simulink model "hex_simplify_control"  (R2017a)
settings: Solver=VariableStepAuto  StartTime=0.0  StopTime=2  RelTol=1e-3
model workspace: external: MATLAB File C:\Users\laure\Documents\Gonzalo\Robotica-II\hexapod-robot\simscape\simplify_model\hex_DataFile1.m (data not in the file)
undefined symbols (not defined in the file): qdd_1, qdd_2, qdd_3, sample_frequency, smiData, X, Y, Z
libraries: sm_lib x20, nesl_utility x19
settings Model: Creator=laure  LastModifiedBy=laure

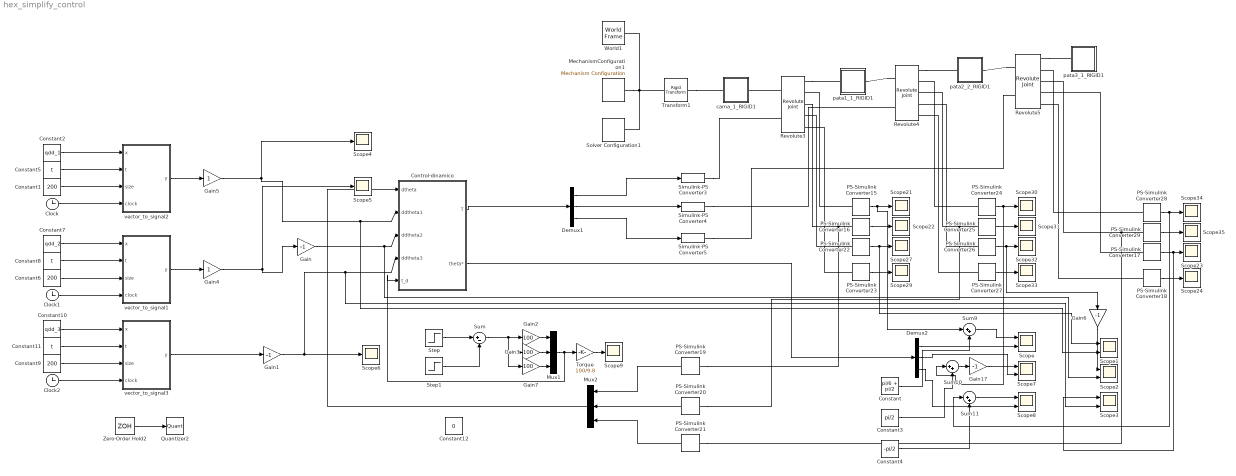
== system hex_simplify_control ==
  Clock : Clock
  Clock1 : Clock
  Clock2 : Clock
  Constant : Constant  Value=pi/6 + pi/2
  Constant1 : Constant  Value=200
  Constant10 : Constant  Value=qdd_3
  Constant11 : Constant  Value=t
  Constant12 : Constant  Value=0
  Constant2 : Constant  Value=qdd_1
  Constant3 : Constant  Value=pi/2
  Constant4 : Constant  Value=-pi/2
  Constant5 : Constant  Value=t
  Constant6 : Constant  Value=200
  Constant7 : Constant  Value=qdd_2
  Constant8 : Constant  Value=t
  Constant9 : Constant  Value=200
  Control-dinamico : Subsystem
  Demux1 : Demux  Outputs=3
  Demux2 : Demux  Outputs=3
  Gain{,1,6,17} (4 alike) : Gain  Gain=-1
  Gain2 : Gain  Gain=100
  Gain3 : Gain  Gain=100
  Gain4 : Gain
  Gain5 : Gain
  Gain7 : Gain  Gain=100
  MechanismConfiguration1 : sm_lib/Utilities/Mechanism Configuration  UniformGravity=Constant  GravityVector=[0 0 -9.81]  GravityUnits=m/s^2  LinearizationDelta=0.001
  Mux1 : Mux  Inputs=3
  Mux2 : Mux  Inputs=3
  PS-Simulink Converter{15..29} (15 alike) : nesl_utility/PS-Simulink Converter  PhysicalDomain=network_engine_domain  SubClassName=ps_output  LeftPortType=input  RightPortType=output  PseudoPeriodic=off  Frequencies=[]  Unit=1  AffineConversion=off
  Quantizer2 : Quantizer  QuantizationInterval=1/sample_frequency
  Revolute3 : sm_lib/Joints/Revolute Joint  SenseConstraintForce=off  SenseConstraintForceX=off  SenseConstraintForceY=off  SenseConstraintForceZ=off  SenseConstraintTorque=off  SenseConstraintTorqueX=off  SenseConstraintTorqueY=off  SenseConstraintTorqueZ=off  SenseTotalForce=off  SenseTotalForceX=off  SenseTotalForceY=off  SenseTotalForceZ=off  SenseTotalTorque=off  SenseTotalTorqueX=off  SenseTotalTorqueY=off  SenseTotalTorqueZ=off  CompositeWrenchDir=FollowerOnBase  CompositeWrenchFrame=BaseFrame  EquilibriumPosition=0  EquilibriumPositionUnits=rad  SpringStiffness=0  SpringStiffnessUnits=N*m/rad  DampingCoefficient=0.1  DampingCoefficientUnits=N*m/(rad/s)  TorqueActuationMode=InputTorque  MotionActuationMode=ComputedMotion  SensePosition=on  SenseVelocity=on  SenseAcceleration=on  SenseTorqueForce=on  PositionTargetSpecify=on  PositionTargetPriority=Low  PositionTargetValue=-pi/2 - pi/6  PositionTargetValueUnits=rad  VelocityTargetSpecify=off  VelocityTargetPriority=High  VelocityTargetValue=0  VelocityTargetValueUnits=deg/s
  Revolute4 : sm_lib/Joints/Revolute Joint  SenseConstraintForce=off  SenseConstraintForceX=off  SenseConstraintForceY=off  SenseConstraintForceZ=off  SenseConstraintTorque=off  SenseConstraintTorqueX=off  SenseConstraintTorqueY=off  SenseConstraintTorqueZ=off  SenseTotalForce=off  SenseTotalForceX=off  SenseTotalForceY=off  SenseTotalForceZ=off  SenseTotalTorque=off  SenseTotalTorqueX=off  SenseTotalTorqueY=off  SenseTotalTorqueZ=off  CompositeWrenchDir=FollowerOnBase  CompositeWrenchFrame=BaseFrame  EquilibriumPosition=0  EquilibriumPositionUnits=rad  SpringStiffness=0  SpringStiffnessUnits=N*m/rad  DampingCoefficient=0.1  DampingCoefficientUnits=N*m/(rad/s)  TorqueActuationMode=InputTorque  MotionActuationMode=ComputedMotion  SensePosition=on  SenseVelocity=on  SenseAcceleration=on  SenseTorqueForce=on  PositionTargetSpecify=on  PositionTargetPriority=Low  PositionTargetValue=-pi/2  PositionTargetValueUnits=rad  VelocityTargetSpecify=on  VelocityTargetPriority=High  VelocityTargetValue=0  VelocityTargetValueUnits=deg/s
  Revolute5 : sm_lib/Joints/Revolute Joint  SenseConstraintForce=off  SenseConstraintForceX=off  SenseConstraintForceY=off  SenseConstraintForceZ=off  SenseConstraintTorque=off  SenseConstraintTorqueX=off  SenseConstraintTorqueY=off  SenseConstraintTorqueZ=off  SenseTotalForce=off  SenseTotalForceX=off  SenseTotalForceY=off  SenseTotalForceZ=off  SenseTotalTorque=off  SenseTotalTorqueX=off  SenseTotalTorqueY=off  SenseTotalTorqueZ=off  CompositeWrenchDir=FollowerOnBase  CompositeWrenchFrame=BaseFrame  EquilibriumPosition=0  EquilibriumPositionUnits=rad  SpringStiffness=0  SpringStiffnessUnits=N*m/rad  DampingCoefficient=0.1  DampingCoefficientUnits=N*m/(rad/s)  TorqueActuationMode=InputTorque  MotionActuationMode=ComputedMotion  SensePosition=on  SenseVelocity=on  SenseAcceleration=on  SenseTorqueForce=on  PositionTargetSpecify=on  PositionTargetPriority=Low  PositionTargetValue=0  PositionTargetValueUnits=rad  VelocityTargetSpecify=off  VelocityTargetPriority=High  VelocityTargetValue=0  VelocityTargetValueUnits=deg/s
  Scope{,1..3,7..8} (6 alike) : Scope  NumInputPorts=2
  Scope{4..6,9,21..24,27,29..35} (16 alike) : Scope
  Simulink-PS Converter3 : nesl_utility/Simulink-PS Converter  PhysicalDomain=network_engine_domain  SubClassName=ps_input  LeftPortType=input  RightPortType=output  PseudoPeriodic=off  Frequencies=[]  NoiseDistribution=none  NoiseParameters=[]  Unit=1  AffineConversion=off  FilteringAndDerivatives=filter  SimscapeFilterOrder=2  InputFilterTimeConstant=0.001  UdotUserProvided=0
  Simulink-PS Converter4 : nesl_utility/Simulink-PS Converter  PhysicalDomain=network_engine_domain  SubClassName=ps_input  LeftPortType=input  RightPortType=output  PseudoPeriodic=off  Frequencies=[]  NoiseDistribution=none  NoiseParameters=[]  Unit=1  AffineConversion=off  FilteringAndDerivatives=filter  SimscapeFilterOrder=2  InputFilterTimeConstant=0.001  UdotUserProvided=0
  Simulink-PS Converter5 : nesl_utility/Simulink-PS Converter  PhysicalDomain=network_engine_domain  SubClassName=ps_input  LeftPortType=input  RightPortType=output  PseudoPeriodic=off  Frequencies=[]  NoiseDistribution=none  NoiseParameters=[]  Unit=1  AffineConversion=off  FilteringAndDerivatives=filter  SimscapeFilterOrder=2  InputFilterTimeConstant=0.001  UdotUserProvided=0
  Solver Configuration1 : nesl_utility/Solver Configuration  PhysicalDomain=network_engine_domain  SubClassName=solver  LeftPortType=input  RightPortType=generic  Accelerate=off  Tones=[]  Harmonics=[]  SimulateNoise=off  Profile=off  UseLocalSampling=off  EnableSwitchedLinearOptims=on  FrequencyDomain=off  UseCCode=off  RelTol=0.001  AbsTol=1e-06  MinStep=1e-09  ToWorkspace=off  RevertToSquareIcSolve=off  NumHomotopyIterations=100  PhasorMode=off  PhasorModeNumHarmonics=1  OverrideAbsTol=off  DoDC=off  ResidualTolerance=1e-09  UseLocalSolver=off  LocalSolverChoice=NE_BACKWARD_EULER_ADVANCER  LocalSolverSampleTime=0.001  DoFixedCost=off  MaxNonlinIter=3  MaxModeIter=2  LinearAlgebra=Sparse  DelaysMemoryBudget=1024  AutomaticFiltering=on  FilteringTimeConstant=0.001
  Step : Step  Time=0.1  After=0.01  SampleTime=0
  Step1 : Step  After=0.01  SampleTime=0
  Sum : Sum  Inputs=|+-
  Sum10 : Sum  Inputs=|++
  Sum11 : Sum  Inputs=|++
  Sum9 : Sum  Inputs=|++
  Torque : Gain  Gain=100/9.8
  Transform1 : sm_lib/Frames and Transforms/Rigid Transform  TranslationMethod=Cartesian  TranslationStandardOffset=0  TranslationLengthUnit=mm  TranslationStandardAxis=+Z  TranslationCartesianOffset=smiData.RigidTransform(7).translation  TranslationROffset=0  TranslationROffsetUnits=m  TranslationZOffset=0  TranslationZOffsetUnits=m  TranslationThetaOffset=0  TranslationThetaOffsetUnits=deg  RotationMethod=ArbitraryAxis  RotationAngleUnits=rad  RotationStandardAxis=+Z  RotationAngle=smiData.RigidTransform(7).angle  RotationArbitraryAxis=smiData.RigidTransform(7).axis  FollAlignAxisA=+X  BaseAlignAxisA=+Y  FollAlignAxisB=+Y  BaseAlignAxisB=+Z  RotationSequenceAxes=FollowerAxes  RotationSequence=XYX  RotationSequenceAngles=[0 0 0]  RotationSequenceAnglesUnits=deg  RotationMatrix=[1 0 0; 0 1 0; 0 0 1]
  World1 : sm_lib/Frames and Transforms/World Frame
  Zero-Order Hold2 : ZeroOrderHold  SampleTime=1/sample_frequency
  cama_1_RIGID1 : Subsystem
  pata1_1_RIGID1 : Subsystem
  pata2_2_RIGID1 : Subsystem
  pata3_1_RIGID1 : Subsystem
  vector_to_signal1 : Subsystem
  vector_to_signal2 : Subsystem
  vector_to_signal3 : Subsystem
  wires:
  PS-Simulink Converter26/1 -> Gain6/1, Scope32/1
  PS-Simulink Converter29/1 -> Scope35/1
  PS-Simulink Converter24/1 -> Sum10/1, Scope30/1
  PS-Simulink Converter18/1 -> Scope24/1
  PS-Simulink Converter23/1 -> Scope29/1
  PS-Simulink Converter27/1 -> Scope33/1
  Demux2/2 -> Scope7/2
  PS-Simulink Converter22/1 -> Scope1/1, Scope27/1
  PS-Simulink Converter20/1 -> Mux2/2
  Demux1/2 -> Simulink-PS Converter4/1
  PS-Simulink Converter19/1 -> Mux2/1
  Demux1/1 -> Simulink-PS Converter3/1
  PS-Simulink Converter15/1 -> Sum9/1, Scope21/1
  Demux1/3 -> Simulink-PS Converter5/1
  PS-Simulink Converter25/1 -> Scope31/1
  Demux2/3 -> Scope8/2
  PS-Simulink Converter21/1 -> Mux2/3
  PS-Simulink Converter16/1 -> Scope22/1
  Demux2/1 -> Scope/2
  PS-Simulink Converter28/1 -> Sum11/1, Scope34/1
  Sum9/1 -> Scope/1
  Sum10/1 -> Gain17/1
  Sum11/1 -> Scope8/1
  Constant/1 -> Sum9/2
  Constant4/1 -> Sum11/2
  Constant3/1 -> Sum10/2
  Gain17/1 -> Scope7/1
  Mux2/1 -> Control-dinamico/1(dtheta)
  Control-dinamico/1(T) -> Demux1/1
  Control-dinamico/2(theta*) -> Demux2/1
  Gain6/1 -> Scope2/1
  Clock/1 -> vector_to_signal2/4("clock ")
  Constant1/1 -> vector_to_signal2/3(size)
  Constant5/1 -> vector_to_signal2/2(t)
  Constant2/1 -> vector_to_signal2/1(x)
  Constant6/1 -> vector_to_signal1/3(size)
  Clock1/1 -> vector_to_signal1/4("clock ")
  Constant7/1 -> vector_to_signal1/1(x)
  Constant8/1 -> vector_to_signal1/2(t)
  Constant10/1 -> vector_to_signal3/1(x)
  Constant11/1 -> vector_to_signal3/2(t)
  Clock2/1 -> vector_to_signal3/4("clock ")
  Constant9/1 -> vector_to_signal3/3(size)
  Gain/1 -> Scope2/2, Control-dinamico/3(ddtheta2)
  Gain1/1 -> Scope6/1, Scope3/2, Control-dinamico/4(ddtheta3)
  Mux1/1 -> Torque/1, Control-dinamico/5(t_d)
  Step/1 -> Sum/1
  Step1/1 -> Sum/2
  Gain2/1 -> Mux1/1
  Gain3/1 -> Mux1/2
  Zero-Order Hold2/1 -> Quantizer2/1
  Gain4/1 -> Gain/1, Scope5/1
  Gain5/1 -> Scope1/2, Control-dinamico/2(ddtheta1), Scope4/1
  Sum/1 -> Gain2/1, Gain7/1, Gain3/1
  Gain7/1 -> Mux1/3
  vector_to_signal3/1(y) -> Gain1/1
  PS-Simulink Converter17/1 -> Scope3/1, Scope23/1
  vector_to_signal1/1(y) -> Gain4/1
  vector_to_signal2/1(y) -> Gain5/1
  Torque/1 -> Scope9/1
  connections:
  Revolute4/RConn3 -- PS-Simulink Converter25/LConn1 -- PS-Simulink Converter20/LConn1
  PS-Simulink Converter16/LConn1 -- Revolute3/RConn3 -- PS-Simulink Converter19/LConn1
  PS-Simulink Converter28/LConn1 -- Revolute5/RConn2
  Solver Configuration1/RConn1 -- MechanismConfiguration1/RConn1 -- World1/RConn1 -- Transform1/LConn1
  Revolute3/RConn1 -- pata1_1_RIGID1/LConn1
  PS-Simulink Converter15/LConn1 -- Revolute3/RConn2
  PS-Simulink Converter29/LConn1 -- PS-Simulink Converter21/LConn1 -- Revolute5/RConn3
  PS-Simulink Converter23/LConn1 -- Revolute3/RConn5
  Transform1/RConn1 -- cama_1_RIGID1/LConn1
  PS-Simulink Converter22/LConn1 -- Revolute3/RConn4
  PS-Simulink Converter26/LConn1 -- Revolute4/RConn4
  Revolute4/RConn1 -- pata2_2_RIGID1/LConn1
  PS-Simulink Converter17/LConn1 -- Revolute5/RConn4
  Simulink-PS Converter4/RConn1 -- Revolute4/LConn2
  Revolute3/LConn1 -- cama_1_RIGID1/RConn1
  Revolute5/RConn1 -- pata3_1_RIGID1/LConn1
  Revolute5/LConn1 -- pata2_2_RIGID1/RConn1
  PS-Simulink Converter27/LConn1 -- Revolute4/RConn5
  PS-Simulink Converter24/LConn1 -- Revolute4/RConn2
  PS-Simulink Converter18/LConn1 -- Revolute5/RConn5
  Simulink-PS Converter5/RConn1 -- Revolute5/LConn2
  Revolute4/LConn1 -- pata1_1_RIGID1/RConn1
  Simulink-PS Converter3/RConn1 -- Revolute3/LConn2

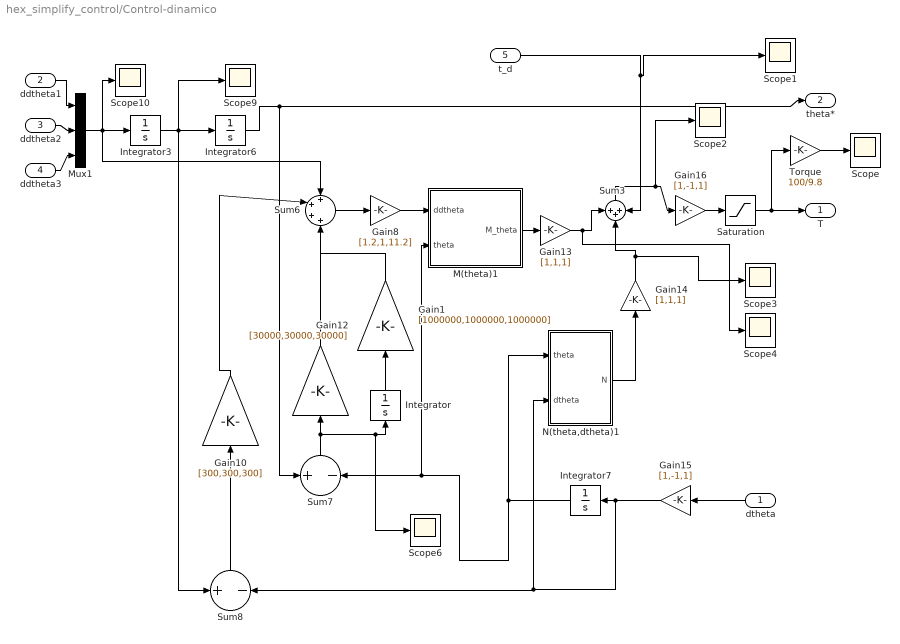
== system hex_simplify_control/Control-dinamico ==
  dtheta : Inport
  ddtheta1 : Inport  Port=2
  ddtheta2 : Inport  Port=3
  ddtheta3 : Inport  Port=4
  t_d : Inport  Port=5
  Gain1 : Gain  Gain=[1000000,1000000,1000000]
  Gain10 : Gain  Gain=[300,300,300]
  Gain12 : Gain  Gain=[30000,30000,30000]
  Gain13 : Gain  Gain=[1,1,1]
  Gain14 : Gain  Gain=[1,1,1]
  Gain15 : Gain  Gain=[1,-1,1]
  Gain16 : Gain  Gain=[1,-1,1]
  Gain8 : Gain  Gain=[1.2,1,11.2]
  Integrator : Integrator  InitialCondition=[0,0,0]
  Integrator3 : Integrator
  Integrator6 : Integrator  InitialCondition=[0,0,-pi/2]
  Integrator7 : Integrator  InitialCondition=[0,0,-pi/2]
  M(theta)1 : Subsystem
  Mux1 : Mux  Inputs=3
  N(theta,dtheta)1 : Subsystem
  Saturation : Saturate  UpperLimit=5  LowerLimit=-5  LinearizeAsGain=off  ZeroCross=off
  Scope{,1..4,6,9..10} (8 alike) : Scope
  Sum3 : Sum  Inputs=+++
  Sum6 : Sum  Inputs=++++
  Sum7 : Sum  Inputs=+-
  Sum8 : Sum  Inputs=+-
  Torque : Gain  Gain=100/9.8
  T : Outport
  theta* : Outport  Port=2
  wires:
  Gain15/1 -> Integrator7/1, N(theta,dtheta)1/2(dtheta), Sum8/2
  Gain16/1 -> Saturation/1
  Saturation/1 -> Torque/1, T/1
  Integrator7/1 -> M(theta)1/2(theta), Sum7/2, N(theta,dtheta)1/1(theta)
  Gain13/1 -> Scope4/1, Sum3/1
  Sum3/1 -> Scope2/1, Gain16/1
  Gain12/1 -> Sum6/3
  N(theta,dtheta)1/1(N) -> Gain14/1
  Sum7/1 -> Integrator/1, Scope6/1, Gain12/1
  Gain10/1 -> Sum6/2
  M(theta)1/1(M_theta) -> Gain13/1
  dtheta/1 -> Gain15/1
  Sum6/1 -> Gain8/1
  Gain14/1 -> Scope3/1, Sum3/2
  Mux1/1 -> Sum6/1, Integrator3/1, Scope10/1
  Integrator6/1 -> theta*/1, Sum7/1
  Integrator3/1 -> Integrator6/1, Sum8/1, Scope9/1
  Sum8/1 -> Gain10/1
  ddtheta1/1 -> Mux1/1
  ddtheta2/1 -> Mux1/2
  ddtheta3/1 -> Mux1/3
  t_d/1 -> Scope1/1, Sum3/3
  Integrator/1 -> Gain1/1
  Gain1/1 -> Sum6/4
  Gain8/1 -> M(theta)1/1(ddtheta)
  Torque/1 -> Scope/1

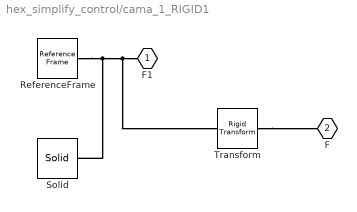
== system hex_simplify_control/cama_1_RIGID1 ==
  ReferenceFrame : sm_lib/Frames and Transforms/Reference Frame
  Solid : sm_lib/Body Elements/Solid  InertiaType=Custom  Mass=smiData.Solid(2).mass  MassUnits=kg  CenterOfMass=smiData.Solid(2).CoM  CenterOfMassUnits=mm  MomentsOfInertia=smiData.Solid(2).MoI  MomentsOfInertiaUnits=kg*mm^2  ProductsOfInertia=smiData.Solid(2).PoI  ProductsOfInertiaUnits=kg*mm^2  DensityBased=on  Density=1000  DensityUnits=kg/m^3  DoExposeReferenceFrame=on  SerializedFrames=<Frames/>  GraphicType=FromGeometry  MarkerShape=Sphere  MarkerSize=10  GraphicVisPropType=SimpleVisualProperties  GraphicDiffuseColor=smiData.Solid(2).color  GraphicSpecularColor=[0.5 0.5 0.5 1.0]  GraphicAmbientColor=[0.15 0.15 0.15 1.0]  GraphicEmissiveColor=[0.0 0.0 0.0 1.0]  GraphicShininess=75  GraphicOpacity=smiData.Solid(2).opacity  GeometryShape=FromFile  RectangleSize=[1 1]  RectangleSizeUnits=m  BrickDimensions=[1 1 1]  BrickDimensionUnits=m  CylinderRadius=1  CylinderRadiusUnits=m  CylinderLength=1  CylinderLengthUnits=m  SphereRadius=1  SphereRadiusUnits=m  EllipsoidRadii=[1 1 1]  EllipsoidRadiiUnits=m  ExtrusionCrossSection=[1 1; -1 1; -1 -1; 1 -1]  ExtrusionCrossSectionUnits=m  ExtrusionLength=1  ExtrusionLengthUnits=m  PolygonNumSides=3  PolygonOuterRadius=1  PolygonOuterRadiusUnits=m  ExtGeomFileType=STEP  ExtGeomFileName=cama_Predeterminado_sldprt.STEP  ExtGeomFileUnits=m  RevolutionCrossSection=[1 1; 1 -1; 2 -1; 2 1]  RevolutionCrossSectionUnits=m  RevolutionExtent=Full  RevolutionAngle=180  RevolutionAngleUnits=deg
  Transform : sm_lib/Frames and Transforms/Rigid Transform  TranslationMethod=Cartesian  TranslationStandardOffset=0  TranslationLengthUnit=mm  TranslationStandardAxis=+Z  TranslationCartesianOffset=smiData.RigidTransform(1).translation  TranslationROffset=0  TranslationROffsetUnits=m  TranslationZOffset=0  TranslationZOffsetUnits=m  TranslationThetaOffset=0  TranslationThetaOffsetUnits=deg  RotationMethod=ArbitraryAxis  RotationAngleUnits=rad  RotationStandardAxis=+Z  RotationAngle=smiData.RigidTransform(1).angle  RotationArbitraryAxis=smiData.RigidTransform(1).axis  FollAlignAxisA=+X  BaseAlignAxisA=+Y  FollAlignAxisB=+Y  BaseAlignAxisB=+Z  RotationSequenceAxes=FollowerAxes  RotationSequence=XYX  RotationSequenceAngles=[0 0 0]  RotationSequenceAnglesUnits=deg  RotationMatrix=[1 0 0; 0 1 0; 0 0 1]
  F1 : PMIOPort  Port=1  Side=Left
  F : PMIOPort  Port=2  Side=Right
  connections:
  Solid/RConn1 -- ReferenceFrame/RConn1 -- Transform/LConn1 -- F1/RConn1
  Transform/RConn1 -- F/RConn1

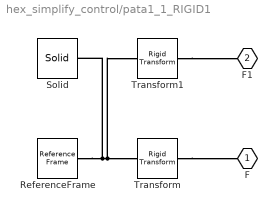
== system hex_simplify_control/pata1_1_RIGID1 ==
  ReferenceFrame : sm_lib/Frames and Transforms/Reference Frame
  Solid : sm_lib/Body Elements/Solid  InertiaType=Custom  Mass=0.133  MassUnits=kg  CenterOfMass=[10+14.1,7.5,-7.5]  CenterOfMassUnits=mm  MomentsOfInertia=[0,0,0]  MomentsOfInertiaUnits=kg*mm^2  ProductsOfInertia=[0,0,0]  ProductsOfInertiaUnits=kg*mm^2  DensityBased=on  Density=1000  DensityUnits=kg/m^3  DoExposeReferenceFrame=on  SerializedFrames=<Frames/>  GraphicType=FromGeometry  MarkerShape=Sphere  MarkerSize=10  GraphicVisPropType=SimpleVisualProperties  GraphicDiffuseColor=smiData.Solid(4).color  GraphicSpecularColor=[0.5 0.5 0.5 1.0]  GraphicAmbientColor=[0.15 0.15 0.15 1.0]  GraphicEmissiveColor=[0.0 0.0 0.0 1.0]  GraphicShininess=75  GraphicOpacity=smiData.Solid(4).opacity  GeometryShape=FromFile  RectangleSize=[1 1]  RectangleSizeUnits=m  BrickDimensions=[1 1 1]  BrickDimensionUnits=m  CylinderRadius=1  CylinderRadiusUnits=m  CylinderLength=1  CylinderLengthUnits=m  SphereRadius=1  SphereRadiusUnits=m  EllipsoidRadii=[1 1 1]  EllipsoidRadiiUnits=m  ExtrusionCrossSection=[1 1; -1 1; -1 -1; 1 -1]  ExtrusionCrossSectionUnits=m  ExtrusionLength=1  ExtrusionLengthUnits=m  PolygonNumSides=3  PolygonOuterRadius=1  PolygonOuterRadiusUnits=m  ExtGeomFileType=STEP  ExtGeomFileName=pata1_Predeterminado_sldprt.STEP  ExtGeomFileUnits=m  RevolutionCrossSection=[1 1; 1 -1; 2 -1; 2 1]  RevolutionCrossSectionUnits=m  RevolutionExtent=Full  RevolutionAngle=180  RevolutionAngleUnits=deg
  Transform : sm_lib/Frames and Transforms/Rigid Transform  TranslationMethod=Cartesian  TranslationStandardOffset=0  TranslationLengthUnit=mm  TranslationStandardAxis=+Z  TranslationCartesianOffset=smiData.RigidTransform(2).translation  TranslationROffset=0  TranslationROffsetUnits=m  TranslationZOffset=0  TranslationZOffsetUnits=m  TranslationThetaOffset=0  TranslationThetaOffsetUnits=deg  RotationMethod=ArbitraryAxis  RotationAngleUnits=rad  RotationStandardAxis=+Z  RotationAngle=smiData.RigidTransform(2).angle  RotationArbitraryAxis=smiData.RigidTransform(2).axis  FollAlignAxisA=+X  BaseAlignAxisA=+Y  FollAlignAxisB=+Y  BaseAlignAxisB=+Z  RotationSequenceAxes=FollowerAxes  RotationSequence=XYX  RotationSequenceAngles=[0 0 0]  RotationSequenceAnglesUnits=deg  RotationMatrix=[1 0 0; 0 1 0; 0 0 1]
  Transform1 : sm_lib/Frames and Transforms/Rigid Transform  TranslationMethod=Cartesian  TranslationStandardOffset=0  TranslationLengthUnit=mm  TranslationStandardAxis=+Z  TranslationCartesianOffset=smiData.RigidTransform(3).translation  TranslationROffset=0  TranslationROffsetUnits=m  TranslationZOffset=0  TranslationZOffsetUnits=m  TranslationThetaOffset=0  TranslationThetaOffsetUnits=deg  RotationMethod=ArbitraryAxis  RotationAngleUnits=rad  RotationStandardAxis=+Z  RotationAngle=smiData.RigidTransform(3).angle  RotationArbitraryAxis=smiData.RigidTransform(3).axis  FollAlignAxisA=+X  BaseAlignAxisA=+Y  FollAlignAxisB=+Y  BaseAlignAxisB=+Z  RotationSequenceAxes=FollowerAxes  RotationSequence=XYX  RotationSequenceAngles=[0 0 0]  RotationSequenceAnglesUnits=deg  RotationMatrix=[1 0 0; 0 1 0; 0 0 1]
  F : PMIOPort  Port=1  Side=Left
  F1 : PMIOPort  Port=2  Side=Right
  connections:
  Solid/RConn1 -- ReferenceFrame/RConn1 -- Transform/LConn1 -- Transform1/LConn1
  Transform/RConn1 -- F/RConn1
  Transform1/RConn1 -- F1/RConn1

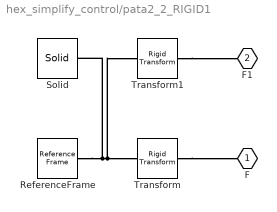
== system hex_simplify_control/pata2_2_RIGID1 ==
  ReferenceFrame : sm_lib/Frames and Transforms/Reference Frame
  Solid : sm_lib/Body Elements/Solid  InertiaType=Custom  Mass=0.013  MassUnits=kg  CenterOfMass=[47.9, 7.5, 12.5]  CenterOfMassUnits=mm  MomentsOfInertia=[0,0,0]  MomentsOfInertiaUnits=kg*mm^2  ProductsOfInertia=[0,0,0]  ProductsOfInertiaUnits=kg*mm^2  DensityBased=on  Density=1000  DensityUnits=kg/m^3  DoExposeReferenceFrame=on  SerializedFrames=<Frames/>  GraphicType=FromGeometry  MarkerShape=Sphere  MarkerSize=10  GraphicVisPropType=SimpleVisualProperties  GraphicDiffuseColor=smiData.Solid(3).color  GraphicSpecularColor=[0.5 0.5 0.5 1.0]  GraphicAmbientColor=[0.15 0.15 0.15 1.0]  GraphicEmissiveColor=[0.0 0.0 0.0 1.0]  GraphicShininess=75  GraphicOpacity=smiData.Solid(3).opacity  GeometryShape=FromFile  RectangleSize=[1 1]  RectangleSizeUnits=m  BrickDimensions=[1 1 1]  BrickDimensionUnits=m  CylinderRadius=1  CylinderRadiusUnits=m  CylinderLength=1  CylinderLengthUnits=m  SphereRadius=1  SphereRadiusUnits=m  EllipsoidRadii=[1 1 1]  EllipsoidRadiiUnits=m  ExtrusionCrossSection=[1 1; -1 1; -1 -1; 1 -1]  ExtrusionCrossSectionUnits=m  ExtrusionLength=1  ExtrusionLengthUnits=m  PolygonNumSides=3  PolygonOuterRadius=1  PolygonOuterRadiusUnits=m  ExtGeomFileType=STEP  ExtGeomFileName=pata2_Predeterminado_sldprt.STEP  ExtGeomFileUnits=m  RevolutionCrossSection=[1 1; 1 -1; 2 -1; 2 1]  RevolutionCrossSectionUnits=m  RevolutionExtent=Full  RevolutionAngle=180  RevolutionAngleUnits=deg
  Transform : sm_lib/Frames and Transforms/Rigid Transform  TranslationMethod=Cartesian  TranslationStandardOffset=0  TranslationLengthUnit=mm  TranslationStandardAxis=+Z  TranslationCartesianOffset=smiData.RigidTransform(4).translation  TranslationROffset=0  TranslationROffsetUnits=m  TranslationZOffset=0  TranslationZOffsetUnits=m  TranslationThetaOffset=0  TranslationThetaOffsetUnits=deg  RotationMethod=ArbitraryAxis  RotationAngleUnits=rad  RotationStandardAxis=+Z  RotationAngle=smiData.RigidTransform(4).angle  RotationArbitraryAxis=smiData.RigidTransform(4).axis  FollAlignAxisA=+X  BaseAlignAxisA=+Y  FollAlignAxisB=+Y  BaseAlignAxisB=+Z  RotationSequenceAxes=FollowerAxes  RotationSequence=XYX  RotationSequenceAngles=[0 0 0]  RotationSequenceAnglesUnits=deg  RotationMatrix=[1 0 0; 0 1 0; 0 0 1]
  Transform1 : sm_lib/Frames and Transforms/Rigid Transform  TranslationMethod=Cartesian  TranslationStandardOffset=0  TranslationLengthUnit=mm  TranslationStandardAxis=+Z  TranslationCartesianOffset=smiData.RigidTransform(5).translation  TranslationROffset=0  TranslationROffsetUnits=m  TranslationZOffset=0  TranslationZOffsetUnits=m  TranslationThetaOffset=0  TranslationThetaOffsetUnits=deg  RotationMethod=ArbitraryAxis  RotationAngleUnits=rad  RotationStandardAxis=+Z  RotationAngle=smiData.RigidTransform(5).angle  RotationArbitraryAxis=smiData.RigidTransform(5).axis  FollAlignAxisA=+X  BaseAlignAxisA=+Y  FollAlignAxisB=+Y  BaseAlignAxisB=+Z  RotationSequenceAxes=FollowerAxes  RotationSequence=XYX  RotationSequenceAngles=[0 0 0]  RotationSequenceAnglesUnits=deg  RotationMatrix=[1 0 0; 0 1 0; 0 0 1]
  F : PMIOPort  Port=1  Side=Left
  F1 : PMIOPort  Port=2  Side=Right
  connections:
  Solid/RConn1 -- ReferenceFrame/RConn1 -- Transform/LConn1 -- Transform1/LConn1
  Transform/RConn1 -- F/RConn1
  Transform1/RConn1 -- F1/RConn1

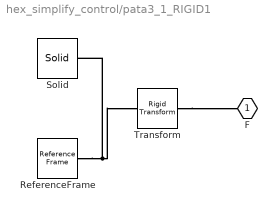
== system hex_simplify_control/pata3_1_RIGID1 ==
  ReferenceFrame : sm_lib/Frames and Transforms/Reference Frame
  Solid : sm_lib/Body Elements/Solid  InertiaType=Custom  Mass=0.083  MassUnits=kg  CenterOfMass=[7.5,7.5,-10-15.57]  CenterOfMassUnits=mm  MomentsOfInertia=[0,0,0]  MomentsOfInertiaUnits=kg*mm^2  ProductsOfInertia=[0,0,0]  ProductsOfInertiaUnits=kg*mm^2  DensityBased=on  Density=1000  DensityUnits=kg/m^3  DoExposeReferenceFrame=on  SerializedFrames=<Frames/>  GraphicType=FromGeometry  MarkerShape=Sphere  MarkerSize=10  GraphicVisPropType=SimpleVisualProperties  GraphicDiffuseColor=smiData.Solid(1).color  GraphicSpecularColor=[0.5 0.5 0.5 1.0]  GraphicAmbientColor=[0.15 0.15 0.15 1.0]  GraphicEmissiveColor=[0.0 0.0 0.0 1.0]  GraphicShininess=75  GraphicOpacity=smiData.Solid(1).opacity  GeometryShape=FromFile  RectangleSize=[1 1]  RectangleSizeUnits=m  BrickDimensions=[1 1 1]  BrickDimensionUnits=m  CylinderRadius=1  CylinderRadiusUnits=m  CylinderLength=1  CylinderLengthUnits=m  SphereRadius=1  SphereRadiusUnits=m  EllipsoidRadii=[1 1 1]  EllipsoidRadiiUnits=m  ExtrusionCrossSection=[1 1; -1 1; -1 -1; 1 -1]  ExtrusionCrossSectionUnits=m  ExtrusionLength=1  ExtrusionLengthUnits=m  PolygonNumSides=3  PolygonOuterRadius=1  PolygonOuterRadiusUnits=m  ExtGeomFileType=STEP  ExtGeomFileName=pata3_Predeterminado_sldprt.STEP  ExtGeomFileUnits=m  RevolutionCrossSection=[1 1; 1 -1; 2 -1; 2 1]  RevolutionCrossSectionUnits=m  RevolutionExtent=Full  RevolutionAngle=180  RevolutionAngleUnits=deg
  Transform : sm_lib/Frames and Transforms/Rigid Transform  TranslationMethod=Cartesian  TranslationStandardOffset=0  TranslationLengthUnit=mm  TranslationStandardAxis=+Z  TranslationCartesianOffset=smiData.RigidTransform(6).translation  TranslationROffset=0  TranslationROffsetUnits=m  TranslationZOffset=0  TranslationZOffsetUnits=m  TranslationThetaOffset=0  TranslationThetaOffsetUnits=deg  RotationMethod=ArbitraryAxis  RotationAngleUnits=rad  RotationStandardAxis=+Z  RotationAngle=smiData.RigidTransform(6).angle  RotationArbitraryAxis=smiData.RigidTransform(6).axis  FollAlignAxisA=+X  BaseAlignAxisA=+Y  FollAlignAxisB=+Y  BaseAlignAxisB=+Z  RotationSequenceAxes=FollowerAxes  RotationSequence=XYX  RotationSequenceAngles=[0 0 0]  RotationSequenceAnglesUnits=deg  RotationMatrix=[1 0 0; 0 1 0; 0 0 1]
  F : PMIOPort  Port=1  Side=Left
  connections:
  Solid/RConn1 -- ReferenceFrame/RConn1 -- Transform/LConn1
  Transform/RConn1 -- F/RConn1

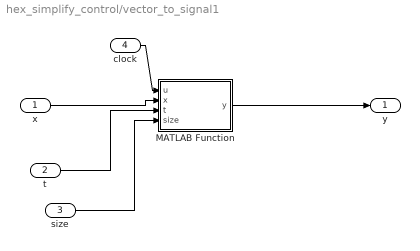
== system hex_simplify_control/vector_to_signal1 ==
  x : Inport
  t : Inport  Port=2
  size : Inport  Port=3
  "clock " : Inport  Port=4
  MATLAB Function : MATLAB Function  TreatAsAtomicUnit=on
  y : Outport
  wires:
  MATLAB Function/1(y) -> y/1
  "clock "/1 -> MATLAB Function/1(u)
  x/1 -> MATLAB Function/2(x)
  t/1 -> MATLAB Function/3(t)
  size/1 -> MATLAB Function/4(size)

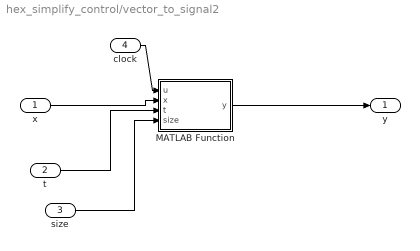
== system hex_simplify_control/vector_to_signal2 ==
  x : Inport
  t : Inport  Port=2
  size : Inport  Port=3
  "clock " : Inport  Port=4
  MATLAB Function : MATLAB Function  TreatAsAtomicUnit=on
  y : Outport
  wires:
  MATLAB Function/1(y) -> y/1
  "clock "/1 -> MATLAB Function/1(u)
  x/1 -> MATLAB Function/2(x)
  t/1 -> MATLAB Function/3(t)
  size/1 -> MATLAB Function/4(size)

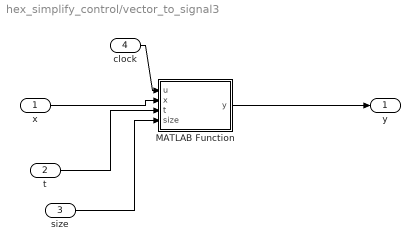
== system hex_simplify_control/vector_to_signal3 ==
  x : Inport
  t : Inport  Port=2
  size : Inport  Port=3
  "clock " : Inport  Port=4
  MATLAB Function : MATLAB Function  TreatAsAtomicUnit=on
  y : Outport
  wires:
  MATLAB Function/1(y) -> y/1
  "clock "/1 -> MATLAB Function/1(u)
  x/1 -> MATLAB Function/2(x)
  t/1 -> MATLAB Function/3(t)
  size/1 -> MATLAB Function/4(size)

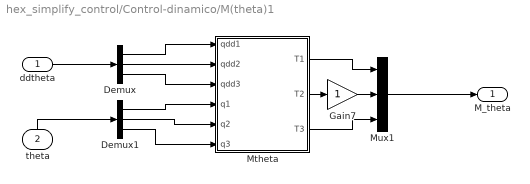
== system hex_simplify_control/Control-dinamico/M(theta)1 ==
  ddtheta : Inport
  theta : Inport  Port=2
  Demux : Demux  Outputs=3
  Demux1 : Demux  Outputs=3
  Gain7 : Gain
  Mtheta : MATLAB Function  TreatAsAtomicUnit=on
  Mux1 : Mux  Inputs=3
  M_theta : Outport
  wires:
  Mux1/1 -> M_theta/1
  Mtheta/3(T3) -> Mux1/3
  Mtheta/2(T2) -> Gain7/1
  Mtheta/1(T1) -> Mux1/1
  Gain7/1 -> Mux1/2
  ddtheta/1 -> Demux/1
  theta/1 -> Demux1/1
  Demux/2 -> Mtheta/2(qdd2)
  Demux/1 -> Mtheta/1(qdd1)
  Demux/3 -> Mtheta/3(qdd3)
  Demux1/1 -> Mtheta/4(q1)
  Demux1/2 -> Mtheta/5(q2)
  Demux1/3 -> Mtheta/6(q3)

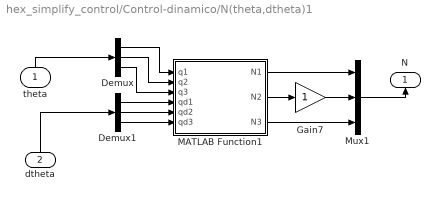
== system hex_simplify_control/Control-dinamico/N(theta,dtheta)1 ==
  theta : Inport
  dtheta : Inport  Port=2
  Demux : Demux  Outputs=3
  Demux1 : Demux  Outputs=3
  Gain7 : Gain
  MATLAB Function1 : MATLAB Function  TreatAsAtomicUnit=on
  Mux1 : Mux  Inputs=3
  N : Outport
  wires:
  MATLAB Function1/3(N3) -> Mux1/3
  MATLAB Function1/1(N1) -> Mux1/1
  Mux1/1 -> N/1
  MATLAB Function1/2(N2) -> Gain7/1
  theta/1 -> Demux/1
  dtheta/1 -> Demux1/1
  Demux/1 -> MATLAB Function1/1(q1)
  Demux/2 -> MATLAB Function1/2(q2)
  Demux/3 -> MATLAB Function1/3(q3)
  Demux1/1 -> MATLAB Function1/4(qd1)
  Demux1/2 -> MATLAB Function1/5(qd2)
  Demux1/3 -> MATLAB Function1/6(qd3)
  Gain7/1 -> Mux1/2

== matlab function hex_simplify_control/vector_to_signal1/MATLAB Function ==
  data: u input; y output; x input; t input; size input
function y = fcn(u, x, t, size)
minor = 1;
y = 0;
for i = 1:size
    if u < t(i)
        minor = i-1;
        break;
    end
end
if u < t(1)
    y = x(1);
elseif u > t(size)
    y = x(5);
else
    y = x(minor) + (x(minor+1)-x(minor))/(t(minor+1)-t(minor))*(u-t(minor));
end

== matlab function hex_simplify_control/vector_to_signal3/MATLAB Function ==
  data: u input; y output; x input; t input; size input
function y = fcn(u, x, t, size)
minor = 1;
y = 0;
for i = 1:size
    if u < t(i)
        minor = i-1;
        break;
    end
end
if u < t(1)
    y = x(1);
elseif u > t(size)
    y = x(5);
else
    y = x(minor) + (x(minor+1)-x(minor))/(t(minor+1)-t(minor))*(u-t(minor));
end

== matlab function hex_simplify_control/Control-dinamico/M(theta)1/Mtheta ==
  data: qdd1 input; T1 output; qdd2 input; T2 output; T3 output; qdd3 input; q1 input; q2 input; q3 input
function [T1, T2, T3] = fcn(qdd1,qdd2,qdd3,q1,q2,q3)

l1 = 0.0285; l2 = 0.0758; l3 = 0.1298;
lc1 = 0.01413; lc2 = l2/2; lc3 = 0.01557;

Ixx1 = 0.000; Ixx2 = 0.000; Ixx3 = 0.000;
Iyy1 = 0.000; Iyy2 = 0.000; Iyy3 = 0.000;
Izz1 = 0.000; Izz2 = 0.000; Izz3 = 0.0000;

gx = 0;
gy = 0;
gz = 9.81;
m1 = 0.133; m2 = 0.013; m3 = 0.083;

Fx = 0;
Fy = 0;
Fz = 0;
b1 = 0.1; b2 = 0.1; b3 = 0.1; 



M = [ Ixx2/2 + Ixx3/2 + Iyy1 + Iyy2/2 + Iyy3/2 - (Ixx3*cos(2*q2 + 2*q3))/2 + (Iyy3*cos(2*q2 + 2*q3))/2 + l1^2*m2 + l1^2*m3 + (l2^2*m3)/2 + lc1^2*m1 + (lc2^2*m2)/2 + (lc3^2*m3)/2 - (Ixx2*cos(2*q2))/2 + (Iyy2*cos(2*q2))/2 + (l2^2*m3*cos(2*q2))/2 + (lc2^2*m2*cos(2*q2))/2 + (lc3^2*m3*cos(2*q2 + 2*q3))/2 + 2*l1*lc3*m3*cos(q2 + q3) + 2*l1*l2*m3*cos(q2) + 2*l1*lc2*m2*cos(q2) + l2*lc3*m3*cos(q3) + l2*lc3*m3*cos(2*q2 + q3),                                                                 0,                                0;
                                                                                                                                                                                                                                                                                                                                                                                                                           0, m3*l2^2 + 2*m3*cos(q3)*l2*lc3 + m2*lc2^2 + m3*lc3^2 + Izz2 + Izz3, Izz3 + lc3*m3*(lc3 + l2*cos(q3));

                                                                                                                                                                                                                                                                                                                                                                                                                           0,                               m3*lc3^2 + l2*m3*cos(q3)*lc3 + Izz3,                  m3*lc3^2 + Izz3];

                                                                                                                                                                                                                                                                                                                                                                                                                       
 T1 = M(1, 1) * qdd1 + M(1, 2) * qdd2 + M(1, 3) * qdd3;
 T2 = M(2, 1) * qdd1 + M(2, 2) * qdd2 + M(2, 3) * qdd3;
 T3 = M(3, 1) * qdd1 + M(3, 2) * qdd2 + M(3, 3) * qdd3;

== matlab function hex_simplify_control/Control-dinamico/N(theta,dtheta)1/MATLAB Function1 ==
  data: q1 input; N1 output; q2 input; N2 output; N3 output; q3 input; qd1 input; qd2 input; qd3 input
function [N1, N2, N3] = fcn(q1,q2,q3,qd1,qd2,qd3)

l1 = 0.0285; l2 = 0.0758; l3 = 0.1298;
lc1 = 0.01413; lc2 = l2/2; lc3 = 0.01557;

Ixx1 = 0.000; Ixx2 = 0.000; Ixx3 = 0.000;
Iyy1 = 0.000; Iyy2 = 0.000; Iyy3 = 0.000;
Izz1 = 0.000; Izz2 = 0.000; Izz3 = 0.0000;

gx = 0;
gy = 0;
gz = 9.81;
m1 = 0.133; m2 = 0.013; m3 = 0.083;



Fx = 0;
Fy = 0;
Fz = 0;
b1 = 0.1; b2 = 0.1; b3 = 0.1; 

N1 = - Fz*l1  + b1*qd1 - Fz*l3*cos(q2 + q3) - Fz*l2*cos(q2) + (gy*lc3*m3*cos(q2 - q1 + q3))/2 + (gx*lc3*m3*sin(q2 - q1 + q3))/2 + (gy*l2*m3*cos(q1 + q2))/2 + (gy*lc2*m2*cos(q1 + q2))/2 - (gx*l2*m3*sin(q1 + q2))/2 - (gx*lc2*m2*sin(q1 + q2))/2 + gy*l1*m2*cos(q1) + gy*l1*m3*cos(q1) + gy*lc1*m1*cos(q1) - gx*l1*m2*sin(q1) - gx*l1*m3*sin(q1) - gx*lc1*m1*sin(q1) + (gy*l2*m3*cos(q1 - q2))/2 + (gy*lc2*m2*cos(q1 - q2))/2 - (gx*l2*m3*sin(q1 - q2))/2 - (gx*lc2*m2*sin(q1 - q2))/2 + (gy*lc3*m3*cos(q1 + q2 + q3))/2 - (gx*lc3*m3*sin(q1 + q2 + q3))/2 + Ixx2*qd1*qd2*sin(2*q2) - Iyy2*qd1*qd2*sin(2*q2) + Ixx3*qd1*qd2*sin(2*q2 + 2*q3) + Ixx3*qd1*qd3*sin(2*q2 + 2*q3) - Iyy3*qd1*qd2*sin(2*q2 + 2*q3) - Iyy3*qd1*qd3*sin(2*q2 + 2*q3)  - l2^2*m3*qd1*qd2*sin(2*q2) - lc2^2*m2*qd1*qd2*sin(2*q2)   - lc3^2*m3*qd1*qd2*sin(2*q2 + 2*q3) - lc3^2*m3*qd1*qd3*sin(2*q2 + 2*q3) - 2*l1*lc3*m3*qd1*qd2*sin(q2 + q3) - 2*l1*lc3*m3*qd1*qd3*sin(q2 + q3) - 2*l1*l2*m3*qd1*qd2*sin(q2) - 2*l1*lc2*m2*qd1*qd2*sin(q2) - l2*lc3*m3*qd1*qd3*sin(q3) - 2*l2*lc3*m3*qd1*qd2*sin(2*q2 + q3) - l2*lc3*m3*qd1*qd3*sin(2*q2 + q3);
N2 = Fy*l3 + b2*qd2 - (Ixx2*qd1^2*sin(2*q2))/2 + (Iyy2*qd1^2*sin(2*q2))/2 + Fy*l2*cos(q3) - (Ixx3*qd1^2*sin(2*q2 + 2*q3))/2 + (Iyy3*qd1^2*sin(2*q2 + 2*q3))/2 + Fx*l2*sin(q3) - (gy*lc3*m3*cos(q2 - q1 + q3))/2 - (gx*lc3*m3*sin(q2 - q1 + q3))/2 + (gy*l2*m3*cos(q1 + q2))/2 + (gy*lc2*m2*cos(q1 + q2))/2 + gz*lc3*m3*cos(q2 + q3) - (gx*l2*m3*sin(q1 + q2))/2 - (gx*lc2*m2*sin(q1 + q2))/2 + gz*l2*m3*cos(q2) + gz*lc2*m2*cos(q2) - (gy*l2*m3*cos(q1 - q2))/2 - (gy*lc2*m2*cos(q1 - q2))/2 + (l2^2*m3*qd1^2*sin(2*q2))/2 + (lc2^2*m2*qd1^2*sin(2*q2))/2 + (gx*l2*m3*sin(q1 - q2))/2 + (gx*lc2*m2*sin(q1 - q2))/2 + (gy*lc3*m3*cos(q1 + q2 + q3))/2 - (gx*lc3*m3*sin(q1 + q2 + q3))/2 + (lc3^2*m3*qd1^2*sin(2*q2 + 2*q3))/2 + l1*lc3*m3*qd1^2*sin(q2 + q3) + l1*l2*m3*qd1^2*sin(q2) + l1*lc2*m2*qd1^2*sin(q2) - l2*lc3*m3*qd3^2*sin(q3) + l2*lc3*m3*qd1^2*sin(2*q2 + q3) - 2*l2*lc3*m3*qd2*qd3*sin(q3);
N3 = Fy*l3 + b3*qd3 - (Ixx3*qd1^2*sin(2*q2 + 2*q3))/2 + (Iyy3*qd1^2*sin(2*q2 + 2*q3))/2 - (gy*lc3*m3*cos(q2 - q1 + q3))/2 - (gx*lc3*m3*sin(q2 - q1 + q3))/2 + gz*lc3*m3*cos(q2 + q3) + (gy*lc3*m3*cos(q1 + q2 + q3))/2 - (gx*lc3*m3*sin(q1 + q2 + q3))/2 + (lc3^2*m3*qd1^2*sin(2*q2 + 2*q3))/2 + l1*lc3*m3*qd1^2*sin(q2 + q3) + (l2*lc3*m3*qd1^2*sin(q3))/2 + l2*lc3*m3*qd2^2*sin(q3) + (l2*lc3*m3*qd1^2*sin(2*q2 + q3))/2 ;

== matlab function hex_simplify_control/vector_to_signal2/MATLAB Function ==
  data: u input; y output; x input; t input; size input
function y = fcn(u, x, t, size)
minor = 1;
y = 0;
for i = 1:size
    if u < t(i)
        minor = i-1;
        break;
    end
end
if u < t(1)
    y = x(1);
elseif u > t(size)
    y = x(5);
else
    y = x(minor) + (x(minor+1)-x(minor))/(t(minor+1)-t(minor))*(u-t(minor));
end
